simulink model "ramadan_2022"  (R2021a)
settings: Solver=ode15s  StartTime=0.0  StopTime=10  MaxStep=1e-2  MinStep=1e-20  RelTol=1e-3
StartFcn:
  | tic
StopFcn:
  | toc
  | 
  | 
  | %if GimbalLockFlag
  |  % fprintf(2, 'Almost reached Gimbal Lock of IMU. Simulation stopped.\n')
  | %end
  | 
  | %fprintf('Elapsed time: %4.2f sec (%4.2f%% realtime)\n', a, tout(end)/a*100)
values from neighbouring files (symbols this model uses):
  Balance = pMod(26:29)    [AssignSimulinkParams.m]    (also in assign_parameters.m = param(26:29))
  BalanceTrunkLat = pMod(22:25)    [AssignSimulinkParams.m]    (also in assign_parameters.m = param(22:25))
  BasisStim = pMod(1:11)    [AssignSimulinkParams.m]    (also in assign_parameters.m = param(1:11))
  CompliantLeg = pMod(12:14)    [AssignSimulinkParams.m]    (also in assign_parameters.m = param(12:14))
  CompliantLegLat = pMod(15)    [AssignSimulinkParams.m]    (also in assign_parameters.m = param(15))
  lp1 = 0.45    [nms3D_prep.m]
  lp2 = 0.55    [nms3D_prep.m]
  N = size(x,1)    [cmaes_hg.m]
  PreventKneeOverextension = pMod(16:21)    [AssignSimulinkParams.m]    (also in assign_parameters.m = param(16:21))
  propulsion = pMod(35)    [AssignSimulinkParams.m]    (also in assign_parameters.m = param(35))
  s = x(1:N-1,:).^2 + x(2:N,:).^2    [cmaes_hg.m]
  Target02 = pMod(30)    [AssignSimulinkParams.m]    (also in assign_parameters.m = param(30))
  Target13 = pMod(31:33)    [AssignSimulinkParams.m]    (also in assign_parameters.m = param(31:33))
  theta0 = pMod(34)    [AssignSimulinkParams.m]    (also in assign_parameters.m = param(34))
  WramameiSL_1000 = readmatrix('WSL_1000_Norm_Sigmoid_MSE_cont.csv')    [nms3D_prep.m]
  ZramameiSL_1000 = readmatrix('ZSL_1000_Norm_Sigmoid_MSE_cont.csv')    [nms3D_prep.m]
undefined symbols (not defined in the file or in its folder): ICs, mParams, X, Y, Z
libraries: nesl_utility x110, sm_lib x88, simulink x79, eeGeneralControl x28, robotmaniplib x10, dspinverses x10, robotcorelib x5, dspmathops x3, pid_lib x2, vrlib x1
(part 7 of 9)

== system ramadan_2022/Muscle Actuation Layer/Muscles Left/Muscle Torque Contributions1/Subsystem ==
  F VAS : Inport
  Moment Arm VAS : Inport  Port=2
  F SOL : Inport  Port=3
  Moment Arm SOL : Inport  Port=4
  Constant : Constant  Value=mParams.muscles.FmaxVec(7)
  Constant1 : Constant  Value=mParams.muscles.FmaxVec(10)
  Divide2 : Product  Inputs=*/
  Product{7..8,11..12} (4 alike) : Product
  Sum4 : Sum
  Sum6 : Sum
  "Leg Torque " : Outport
  wires:
  Sum4/1 -> Divide2/2
  Divide2/1 -> "Leg Torque "/1
  Moment Arm SOL/1 -> Product7/1, Product11/2
  Product11/1 -> Sum6/2
  Constant/1 -> Product8/2
  F VAS/1 -> Product12/1
  Moment Arm VAS/1 -> Product8/1, Product12/2
  Product7/1 -> Sum4/2
  F SOL/1 -> Product11/1
  Sum6/1 -> Divide2/1
  Product12/1 -> Sum6/1
  Constant1/1 -> Product7/2
  Product8/1 -> Sum4/1

== system ramadan_2022/Muscle Actuation Layer/Muscles Right/Muscle Dynamics (Vectorized)/BE force-length relation ==
  note: Buffer Elasticity BE
  lce [lopt] : Inport
  Constant1 : Constant  Value=1-mParams.muscles.w
  Math Function : Math  Operator=square  SignedPower=on  SaturateOnIntegerOverflow=on
  Sum4 : Sum  Inputs=|+-  InputSameDT=on  SaturateOnIntegerOverflow=on  OutDataTypeStr=Inherit: Same as first input
  buffer engaged? : simulink/Logic and Bit Operations/Compare To Zero  relop=<  OutDataTypeStr=boolean  ZeroCross=off
  force of buffer elasticity : Product  Inputs=**
  reference strain [lslack] : Constant  Value=mParams.muscles.w/2
  relative strain : Product  Inputs=*/
  fbe [Fmax] : Outport  VectorParamsAs1DForOutWhenUnconnected=off
  wires:
  force of buffer elasticity/1 -> fbe [Fmax]/1
  Math Function/1 -> force of buffer elasticity/2
  buffer engaged?/1 -> force of buffer elasticity/1
  Constant1/1 -> Sum4/2
  Sum4/1 -> relative strain/1, buffer engaged?/1
  reference strain [lslack]/1 -> relative strain/2
  relative strain/1 -> Math Function/1
  lce [lopt]/1 -> Sum4/1

== system ramadan_2022/Muscle Actuation Layer/Muscles Right/Muscle Dynamics (Vectorized)/CE force-length relation ==
  note: CE Force-Length Relationship
  lce [lopt] : Inport
  Abs : Abs  ZeroCross=off
  Constant1 : Constant
  Constant2 : Constant  Value=3
  Gain : Gain  Gain=log(mParams.muscles.c)
  Math Function : Math  SignedPower=on  SaturateOnIntegerOverflow=on
  Math Function1 : Math  Operator=pow  SignedPower=on  SaturateOnIntegerOverflow=on
  Sum4 : Sum  Inputs=|+-  InputSameDT=on  SaturateOnIntegerOverflow=on  OutDataTypeStr=Inherit: Same as first input
  normalized position : Product  Inputs=*/
  relative width : Constant  Value=mParams.muscles.w
  fce [Fmax] : Outport  VectorParamsAs1DForOutWhenUnconnected=off
  wires:
  Math Function/1 -> fce [Fmax]/1
  Gain/1 -> Math Function/1
  Math Function1/1 -> Gain/1
  Constant2/1 -> Math Function1/2
  normalized position/1 -> Math Function1/1
  Abs/1 -> normalized position/1
  Sum4/1 -> Abs/1
  Constant1/1 -> Sum4/2
  relative width/1 -> normalized position/2
  lce [lopt]/1 -> Sum4/1

== system ramadan_2022/Muscle Actuation Layer/Muscles Right/Muscle Dynamics (Vectorized)/CE inverse force-velocity relation ==
  note: CE Inverse Force-Velocity Relationship
  Fv[Fmax] : Inport
  1 : Product  Inputs=/*
  Constant{1,3..4,8} (4 alike) : Constant
  Constant2 : Constant  Value=mParams.muscles.N
  Curvature : Gain  Gain=mParams.muscles.K  SaturateOnIntegerOverflow=on  OutDataTypeStr=Inherit: Same as input  ParamDataTypeStr=Inherit: Same as input
  Curvature1 : Gain  Gain=7.56*mParams.muscles.K  SaturateOnIntegerOverflow=on  OutDataTypeStr=Inherit: Same as input  ParamDataTypeStr=Inherit: Same as input
  Logical Operator : Logic  Operator=NOT  AllPortsSameDT=off  OutDataTypeStr=boolean
  Logical Operator1 : Logic  Operator=NOT  AllPortsSameDT=off  OutDataTypeStr=boolean
  Slope : Gain  Gain=1e-2  SaturateOnIntegerOverflow=on  OutDataTypeStr=Inherit: Same as input  ParamDataTypeStr=Inherit: Same as input
  Sum1 : Sum  Inputs=|++  InputSameDT=on  SaturateOnIntegerOverflow=on  OutDataTypeStr=Inherit: Same as first input
  Sum2 : Sum  InputSameDT=on  SaturateOnIntegerOverflow=on  OutDataTypeStr=Inherit: Same as first input
  Sum3 : Sum  Inputs=++|  InputSameDT=on  SaturateOnIntegerOverflow=on  OutDataTypeStr=Inherit: Same as first input
  Sum4 : Sum  Inputs=|+-  InputSameDT=on  SaturateOnIntegerOverflow=on  OutDataTypeStr=Inherit: Same as first input
  Sum5 : Sum  Inputs=|-+  InputSameDT=on  SaturateOnIntegerOverflow=on  OutDataTypeStr=Inherit: Same as first input
  Sum6 : Sum  Inputs=-+|  InputSameDT=on  SaturateOnIntegerOverflow=on  OutDataTypeStr=Inherit: Same as first input
  Sum7 : Sum  Inputs=|++  InputSameDT=on  SaturateOnIntegerOverflow=on  OutDataTypeStr=Inherit: Same as first input
  Sum8 : Sum  Inputs=+-|  InputSameDT=on  SaturateOnIntegerOverflow=on  OutDataTypeStr=Inherit: Same as first input
  Sum9 : Sum  InputSameDT=on  SaturateOnIntegerOverflow=on  OutDataTypeStr=Inherit: Same as first input
  extension force within bound? : simulink/Logic and Bit Operations/Compare To Constant  relop=<=  const=mParams.muscles.N  OutDataTypeStr=boolean  ZeroCross=off
  force indicating contraction? : simulink/Logic and Bit Operations/Compare To Constant  relop=<=  const=1  OutDataTypeStr=boolean  ZeroCross=off
  v_concentric : Product  Inputs=*/
  v_concentric1 : Product  Inputs=**
  v_excentric <=N 1 : Product  Inputs=***
  v_excentric <N : Product  Inputs=*/
  v_excentric >N : Product  Inputs=**
  v[vmax] : Outport  VectorParamsAs1DForOutWhenUnconnected=off
  wires:
  Sum2/1 -> Sum9/2
  v_excentric <=N 1/1 -> Sum2/1
  Logical Operator1/1 -> v_excentric >N/1
  v_excentric >N/1 -> Sum2/2
  Logical Operator/1 -> v_excentric <=N 1/1
  Fv[Fmax]/1 -> extension force within bound?/1, force indicating contraction?/1, Curvature/1, Sum4/1, Sum6/2
  extension force within bound?/1 -> Logical Operator1/1, v_excentric <=N 1/3
  force indicating contraction?/1 -> Logical Operator/1, v_concentric1/2
  Sum1/1 -> v_excentric >N/2
  v_concentric1/1 -> Sum9/1
  v_excentric <N/1 -> v_excentric <=N 1/2
  Constant3/1 -> Sum5/1
  Sum5/1 -> 1/1
  Constant2/1 -> Sum5/2, Sum6/1
  Sum6/1 -> Slope/1, 1/2
  Constant8/1 -> Sum1/2
  Slope/1 -> Sum1/1
  Sum9/1 -> v[vmax]/1
  v_concentric/1 -> v_concentric1/1
  Sum7/1 -> v_excentric <N/1
  Sum8/1 -> v_excentric <N/2
  Curvature1/1 -> Sum8/2
  Constant4/1 -> Sum8/1, Sum7/2
  1/1 -> Curvature1/1, Sum7/1
  Sum3/1 -> v_concentric/2
  Sum4/1 -> v_concentric/1
  Constant1/1 -> Sum3/1, Sum4/2
  Curvature/1 -> Sum3/2

== system ramadan_2022/Muscle Actuation Layer/Muscles Right/Muscle Dynamics (Vectorized)/PE force-length relation ==
  note: Parallel Elasticity PE
  lce [lopt] : Inport
  Constant3 : Constant
  Math Function2 : Math  Operator=square  SignedPower=on  SaturateOnIntegerOverflow=on
  Sum1 : Sum  Inputs=|+-  InputSameDT=on  SaturateOnIntegerOverflow=on  OutDataTypeStr=Inherit: Same as first input
  force of buffer elasticity : Product  Inputs=**
  parallel elasticity engaged? : simulink/Logic and Bit Operations/Compare To Zero  relop=>  OutDataTypeStr=boolean  ZeroCross=off
  reference strain [lopt] : Constant  Value=mParams.muscles.w
  relative strain : Product  Inputs=*/
  fpe [Fmax] : Outport  VectorParamsAs1DForOutWhenUnconnected=off
  wires:
  parallel elasticity engaged?/1 -> force of buffer elasticity/1
  force of buffer elasticity/1 -> fpe [Fmax]/1
  Math Function2/1 -> force of buffer elasticity/2
  relative strain/1 -> Math Function2/1
  reference strain [lopt]/1 -> relative strain/2
  Sum1/1 -> relative strain/1, parallel elasticity engaged?/1
  Constant3/1 -> Sum1/2
  lce [lopt]/1 -> Sum1/1

== system ramadan_2022/Muscle Actuation Layer/Muscles Right/Muscle Dynamics (Vectorized)/SE force-length relation ==
  note: SE Force-Length Relationship
  lse [lslack] : Inport
  Constant1 : Constant
  Math Function : Math  Operator=square  SignedPower=on  SaturateOnIntegerOverflow=on
  Sum4 : Sum  Inputs=|+-  InputSameDT=on  SaturateOnIntegerOverflow=on  OutDataTypeStr=Inherit: Same as first input
  force above slack length : Product  Inputs=**
  greater than slack length? : simulink/Logic and Bit Operations/Compare To Zero  relop=>  OutDataTypeStr=boolean  ZeroCross=off
  reference strain [lslack] : Constant  Value=mParams.muscles.eref
  relative strain : Product  Inputs=*/
  fse [Fmax] : Outport  VectorParamsAs1DForOutWhenUnconnected=off
  wires:
  force above slack length/1 -> fse [Fmax]/1
  greater than slack length?/1 -> force above slack length/1
  Constant1/1 -> Sum4/2
  Sum4/1 -> relative strain/1, greater than slack length?/1
  relative strain/1 -> Math Function/1
  lse [lslack]/1 -> Sum4/1
  Math Function/1 -> force above slack length/2
  reference strain [lslack]/1 -> relative strain/2

== system ramadan_2022/Muscle Actuation Layer/Muscles Right/Muscle Torque Contributions/Subsystem ==
  F VAS : Inport
  Moment Arm VAS : Inport  Port=2
  F SOL : Inport  Port=3
  Moment Arm SOL : Inport  Port=4
  Constant : Constant  Value=mParams.muscles.FmaxVec(7)
  Constant1 : Constant  Value=mParams.muscles.FmaxVec(10)
  Divide2 : Product  Inputs=*/
  Product{7..8,11..12} (4 alike) : Product
  Sum4 : Sum
  Sum6 : Sum
  "Leg Torque " : Outport
  wires:
  Sum4/1 -> Divide2/2
  Divide2/1 -> "Leg Torque "/1
  Moment Arm SOL/1 -> Product7/1, Product11/2
  Product11/1 -> Sum6/2
  Constant/1 -> Product8/2
  F VAS/1 -> Product12/1
  Moment Arm VAS/1 -> Product8/1, Product12/2
  Product7/1 -> Sum4/2
  F SOL/1 -> Product11/1
  Sum6/1 -> Divide2/1
  Product12/1 -> Sum6/1
  Constant1/1 -> Product7/2
  Product8/1 -> Sum4/1

== system ramadan_2022/Supraspinal Level/Subsystem/Compute positives forces that generate desired torque profiles/Left ==
  Desired Torques : Inport
  Angles : Inport  Port=2
  Constant : Constant  Value=WramameiSL_1000  VectorParams1D=off  SampleTime=-1
  Constant1 : Constant  Value=|
      | [1.666708374023437500e+01
      | -3.333266830444335938e+01]
  Constant2 : Constant  Value=ZramameiSL_1000
  Denorm : Gain  Gain=[2000, 1500, 3000, 1200, 6000, 350, 1500, 4000, 800]
  Matrix Concatenate : Concatenate  Mode=Multidimensional array
  Matrix Concatenate4 : Concatenate  Mode=Multidimensional array  ConcatenateDimension=2
  Matrix Multiply2 : Product  Multiplication=Matrix(*)
  Matrix Multiply3 : Product  Multiplication=Matrix(*)
  Matrix Multiply8 : Product  Multiplication=Matrix(*)
  Multiply : Gain  Gain=1/960
  Multiply2 : Gain  Gain=1/3.0543
  Saturation : Saturate  UpperLimit=inf  LowerLimit=0  ZeroCross=off
  Saturation2 : Saturate  UpperLimit=inf  LowerLimit=0  ZeroCross=off
  Selector : Selector  InputPortWidth=4  IndexOptions=Index vector (dialog)  Indices=[1 3 4]  OutputSizes=1
  Selector1 : Selector  InputPortWidth=4  IndexOptions=Index vector (dialog)  Indices=[3 4]  OutputSizes=1
  Selector8 : Selector  InputPortWidth=4  IndexOptions=Index vector (dialog)  Indices=2  OutputSizes=1
  Transpose3 : Math  Operator=transpose  SaturateOnIntegerOverflow=on
  Transpose9 : Math  Operator=transpose  SaturateOnIntegerOverflow=on
  sigmoid : Subsystem
  Forces : Outport
  wires:
  Desired Torques/1 -> Selector/1, Selector8/1
  Selector1/1 -> Multiply2/1
  Matrix Multiply2/1 -> Saturation/1
  Selector/1 -> Multiply/1
  Constant/1 -> Matrix Multiply3/2
  Constant2/1 -> Matrix Multiply2/2
  Angles/1 -> Selector1/1
  Matrix Multiply8/1 -> Saturation2/1
  Constant1/1 -> Transpose9/1
  Selector8/1 -> Matrix Multiply8/1
  Transpose9/1 -> Matrix Multiply8/2
  Saturation/1 -> Denorm/1
  Matrix Concatenate4/1 -> Forces/1
  Saturation2/1 -> Matrix Concatenate4/1
  Transpose3/1 -> Matrix Multiply3/1
  Matrix Concatenate/1 -> Transpose3/1  "tr"
  Denorm/1 -> Matrix Concatenate4/2
  Multiply/1 -> Matrix Concatenate/1
  Multiply2/1 -> Matrix Concatenate/2
  sigmoid/1(Out1) -> Matrix Multiply2/1
  Matrix Multiply3/1 -> sigmoid/1(In1)

== system ramadan_2022/Supraspinal Level/Subsystem/Compute positives forces that generate desired torque profiles/Right ==
  Desired Torques : Inport
  Angles : Inport  Port=2
  Constant : Constant  Value=WramameiSL_1000  VectorParams1D=off  SampleTime=-1
  Constant1 : Constant  Value=|
      | [1.666708374023437500e+01
      | -3.333266830444335938e+01]
  Constant2 : Constant  Value=ZramameiSL_1000
  Denorm : Gain  Gain=[2000, 1500, 3000, 1200, 6000, 350, 1500, 4000, 800]
  Matrix Concatenate : Concatenate  Mode=Multidimensional array
  Matrix Concatenate4 : Concatenate  Mode=Multidimensional array  ConcatenateDimension=2
  Matrix Multiply2 : Product  Multiplication=Matrix(*)
  Matrix Multiply3 : Product  Multiplication=Matrix(*)
  Matrix Multiply8 : Product  Multiplication=Matrix(*)
  Multiply : Gain  Gain=1/960
  Multiply2 : Gain  Gain=1/3.0543
  Saturation : Saturate  UpperLimit=inf  LowerLimit=0  ZeroCross=off
  Saturation2 : Saturate  UpperLimit=inf  LowerLimit=0  ZeroCross=off
  Selector : Selector  InputPortWidth=4  IndexOptions=Index vector (dialog)  Indices=[1 3 4]  OutputSizes=1
  Selector1 : Selector  InputPortWidth=4  IndexOptions=Index vector (dialog)  Indices=[3 4]  OutputSizes=1
  Selector8 : Selector  InputPortWidth=4  IndexOptions=Index vector (dialog)  Indices=2  OutputSizes=1
  Transpose3 : Math  Operator=transpose  SaturateOnIntegerOverflow=on
  Transpose9 : Math  Operator=transpose  SaturateOnIntegerOverflow=on
  sigmoid : Subsystem
  Forces : Outport
  wires:
  Desired Torques/1 -> Selector/1, Selector8/1
  Selector1/1 -> Multiply2/1
  Matrix Multiply2/1 -> Saturation/1
  Selector/1 -> Multiply/1
  Constant/1 -> Matrix Multiply3/2
  Constant2/1 -> Matrix Multiply2/2
  Angles/1 -> Selector1/1
  Matrix Multiply8/1 -> Saturation2/1
  Constant1/1 -> Transpose9/1
  Selector8/1 -> Matrix Multiply8/1
  Transpose9/1 -> Matrix Multiply8/2
  Saturation/1 -> Denorm/1
  Matrix Concatenate4/1 -> Forces/1
  Saturation2/1 -> Matrix Concatenate4/1
  Transpose3/1 -> Matrix Multiply3/1
  Matrix Concatenate/1 -> Transpose3/1  "tr"
  Denorm/1 -> Matrix Concatenate4/2
  Multiply/1 -> Matrix Concatenate/1
  Multiply2/1 -> Matrix Concatenate/2
  sigmoid/1(Out1) -> Matrix Multiply2/1
  Matrix Multiply3/1 -> sigmoid/1(In1)

== system ramadan_2022/Supraspinal Level/Subsystem/Stance Leg2/Balance Control Equation [Ankle Strategy] ==
  Desired Acceleration (CoM) : Outport
  wires:
  [propulsion] -> Desired Acceleration (CoM)/1

== system ramadan_2022/Supraspinal Level/Subsystem/Stance Leg2/PD-Controller For Saggital Trunk Balance ==
  Gain : Gain  Gain=-1
  Gain1 : Gain  Gain=-1
  Low-Pass Filter (Discrete or Continuous) : eeGeneralControl/Low-Pass Filter (Discrete or Continuous)  K=1  T=0.01  B=inf  A=-inf  init_option=Inherited from block input  x0=0  Ts=0
  Minus : Sum  Inputs=+-
  PID Controller : pid_lib/PID Controller  Controller=PD  Form=Parallel  TimeDomain=Continuous-time  UseExternalTs=off  SampleTime=-1  IntegratorMethod=Forward Euler  FilterMethod=Forward Euler  ControllerParametersSource=internal  P=30  I=0  D=80  UseFilter=on  N=100  TunerSelectOption=Transfer Function Based (PID Tuner App)  ZeroCross=off  InitialConditionSource=internal  InitialConditionForIntegrator=0  InitialConditionForFilter=0  DifferentiatorICPrevScaledInput=0  ExternalReset=none  TrackingMode=off  Kt=1  LimitOutput=off  SatLimitsSource=internal  UpperSaturationLimit=inf  LowerSaturationLimit=-inf  LinearizeAsGain=on  AntiWindupMode=none  Kb=1  POutMin=[]  POutMax=[]  IOutMin=[]  IOutMax=[]  DOutMin=[]  DOutMax=[]  NOutMin=[]  NOutMax=[]  SumOutMin=[]  SumOutMax=[]  SaturationOutMin=[]  SaturationOutMax=[]  PParamMin=[]  PParamMax=[]  IParamMin=[]  IParamMax=[]  DParamMin=[]  DParamMax=[]  NParamMin=[]  NParamMax=[]  KbParamMin=[]  KbParamMax=[]  KtParamMin=[]  KtParamMax=[]  KbOutMin=[]  KbOutMax=[]  KtOutMin=[]  KtOutMax=[]  IntegratorOutMin=[]  IntegratorOutMax=[]  FilterOutMin=[]  FilterOutMax=[]  SumI1OutMin=[]  SumI1OutMax=[]  SumI2OutMin=[]  SumI2OutMax=[]  SumI3OutMin=[]  SumI3OutMax=[]  SumI4OutMin=[]  SumI4OutMax=[]  SumDOutMin=[]  SumDOutMax=[]  DifferentiatorOutMin=[]  DifferentiatorOutMax=[]  FilterDiffOutCoefMin=[]  FilterDiffOutCoefMax=[]  ReciprocalOutMin=[]  ReciprocalOutMax=[]  SumDenOutMin=[]  SumDenOutMax=[]  SumNumOutMin=[]  SumNumOutMax=[]  DivideOutMin=[]  DivideOutMax=[]  UdiffTsProdOutMin=[]  UdiffTsProdOutMax=[]  NTsProdOutMin=[]  NTsProdOutMax=[]  UintegralTsProdOutMin=[]  UintegralTsProdOutMax=[]  UngainTsProdOutMin=[]  UngainTsProdOutMax=[]  IntegratorContinuousStateAttributes=''  IntegratorStateMustResolveToSignalObject=off  IntegratorRTWStateStorageClass=Auto  FilterContinuousStateAttributes=''  FilterStateMustResolveToSignalObject=off  FilterRTWStateStorageClass=Auto  ParallelPVariant=InternalParameters  IdealPVariant=Disabled  IVariant=Disabled  DVariant=InternalParameters  IntegratorVariant=Disabled  SatVariant=Disabled  AWVariant=Disabled  PCopyVariant=Disabled  TRVariant=Disabled  FdbkBlocksVariant=Forward  IdealPFdbkVariant=Disabled  SatFdbkVariant=Disabled  DerivativeFilterVariant=ContFilter  NVariant=InternalParameters  NCopyVariant=Disabled  FilterICVariant=InternalICsFilter  IntegratorICVariant=Disabled  ExternalResetVariant=Disabled  TRSumVariant=Passthrough  SumFdbkVariant=Disabled  SumVariant=Sum_PD  TsampFilterVariant=InternalTs  TsampNgainVariant=Passthrough  TsampIntegralVariant=Disabled_SignalSpec  ExternalSaturationOutDataTypeStr=Inherit: Same as second input
  To Workspace6 : ToWorkspace  VariableName=RotSag  SampleTime=-1
      settings: Save2DSignal=2-D array (concatenate along first dimension)
  PD Input : Outport
  wires:
  Gain/1 -> Low-Pass Filter (Discrete or Continuous)/1
  Minus/1 -> PID Controller/1
  [TrunkRot_sag] -> To Workspace6/1, Minus/1
  PID Controller/1 -> Gain/1
  [theta0] -> Gain1/1
  Gain1/1 -> Minus/2
  Low-Pass Filter (Discrete or Continuous)/1 -> PD Input/1

== system ramadan_2022/Supraspinal Level/Subsystem/Stance Leg2/Stance Leg ==
  left/right : Inport
  Balance Control [Ankle Strategy] : Inport  Port=2
  PD Input : Inport  Port=3
  Foot Orientation Left : Subsystem
  Foot Orientation Right : Subsystem
  Inverse Dynamics Left Leg : Subsystem
  Mux : Mux  Inputs=2
  Mux1 : Mux  Inputs=2
  NOT2 : Logic  Operator=NOT  AllPortsSameDT=off  OutDataTypeStr=boolean
  Selector : Selector  InputPortWidth=4  IndexOptions=Index vector (dialog)  Indices=[ 4 3 2 1]  OutputSizes=1
  Selector1 : Selector  InputPortWidth=4  IndexOptions=Index vector (dialog)  Indices=[ 4 3 2 1]  OutputSizes=1
  Subsystem : Subsystem
  Transpose : Math  Operator=transpose  SaturateOnIntegerOverflow=on
  long delay 1 : eeGeneralControl/Low-Pass Filter (Discrete or Continuous)  K=1  T=mParams.control.delays.long  B=inf  A=-inf  init_option=Inherited from block input  x0=0  Ts=-1
  long delay 2 : eeGeneralControl/Low-Pass Filter (Discrete or Continuous)  K=1  T=mParams.control.delays.long  B=inf  A=-inf  init_option=Inherited from block input  x0=0  Ts=-1
  long delay 4 : eeGeneralControl/Low-Pass Filter (Discrete or Continuous)  K=1  T=mParams.control.delays.long  B=inf  A=-inf  init_option=Inherited from block input  x0=0  Ts=-1
  Push Off Left : Outport
  Push-Off Right : Outport  Port=2
  wires:
  [Rlegq] -> long delay 2/1
  Selector/1 -> Mux/2
  Selector1/1 -> Mux1/2
  [R_body] -> long delay 4/1
  left/right/1 -> NOT2/1, Inverse Dynamics Left Leg/2(left/right)
  Transpose/1 -> Foot Orientation Right/1(R Pelvis), Foot Orientation Left/1(R Pelvis)
  Foot Orientation Left/1(Orientation Foot (Z)) -> Mux1/1
  Foot Orientation Right/1(Foot Orientation (Z)) -> Mux/1
  Balance Control [Ankle Strategy]/1 -> Inverse Dynamics Left Leg/3(Task), Subsystem/3(Task)
  Inverse Dynamics Left Leg/1(Push-Off (Left)) -> Push Off Left/1
  Mux/1 -> Subsystem/1(Config [5])
  NOT2/1 -> Subsystem/2(left/right)
  Subsystem/1(Push-Off (Right)) -> Push-Off Right/1
  Mux1/1 -> Inverse Dynamics Left Leg/1(Config [5])
  long delay 1/1 -> Selector1/1
  long delay 2/1 -> Selector/1
  long delay 4/1 -> Transpose/1
  [Llegq] -> long delay 1/1
  PD Input/1 -> Subsystem/4(PD Input), Inverse Dynamics Left Leg/4(PD Input)

== system ramadan_2022/Supraspinal Level/Subsystem/Swing Leg/Check Quality Minimal Jerk ==
  In1 : Inport
  In2 : Inport  Port=2
  In3 : Inport  Port=3
  In4 : Inport  Port=4
  Mux1 : Mux
  Mux2 : Mux
  Scope : Scope  NumInputPorts=2
  Scope1 : Scope  NumInputPorts=2
  Selector{1..4} (4 alike) : Selector  InputPortWidth=3  IndexOptions=Index vector (dialog)  Indices=[ 3]  OutputSizes=1
  Selector{5..8} (4 alike) : Selector  InputPortWidth=3  IndexOptions=Index vector (dialog)  Indices=[ 1]  OutputSizes=1
  wires:
  Selector5/1 -> Mux2/1
  Selector1/1 -> Mux1/1
  Mux2/1 -> Scope1/2
  Mux1/1 -> Scope/2
  In1/1 -> Selector5/1, Selector1/1
  Selector8/1 -> Mux2/4
  [Rlegddq] -> Scope/1
  Selector3/1 -> Mux1/3
  Selector2/1 -> Mux1/2
  Selector6/1 -> Mux2/2
  In4/1 -> Selector6/1, Selector2/1
  In3/1 -> Selector4/1, Selector8/1
  In2/1 -> Selector3/1, Selector7/1
  [Rlegq] -> Scope1/1
  Selector7/1 -> Mux2/3
  Selector4/1 -> Mux1/4

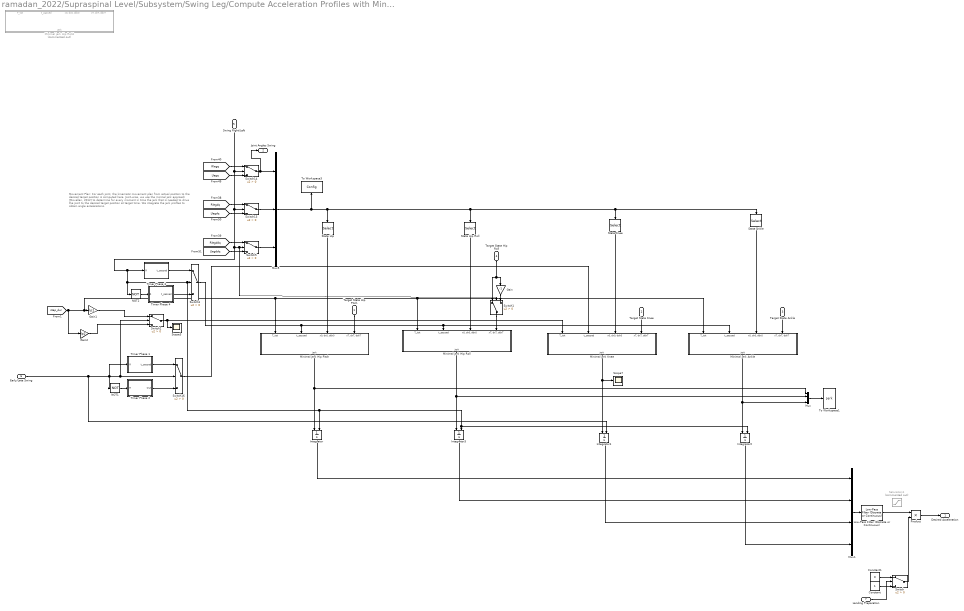
== system ramadan_2022/Supraspinal Level/Subsystem/Swing Leg/Compute Acceleration Profiles with Minimal Jerk Approach ==
  note: Movement Plan: For each joint, the kinematic movement plan from actual position to the desired target position is computed here. Joint-wise, we use the mininal jerk approach [Movellan, 2012] to determine for every moment in time the jerk that is needed to drive the joint to the desired target position at target time. We integrate the jerk profiles to obtain angle accelerations.
  Target State Hip Pitch : Inport
  Target State Knee : Inport  Port=2
  Target State Ankle : Inport  Port=3
  Target State Hip Roll : Inport  Port=4
  Swing Right/Left : Inport  Port=5
  Early/Late Swing : Inport  Port=6
  Landing Preparation : Inport  Port=7
  " Timer Phase 1" : Subsystem
  " Timer Phase 2" : Subsystem
  " Timer Phase 3" : Subsystem
  " Timer Phase 4" : Subsystem
  Constant : Constant
  Constant1 : Constant  Value=0
  Gain : Gain  Gain=-1
  Gain1 : Gain  Gain=lp1
  Gain2 : Gain  Gain=lp2
  Integrator{,1..3} (4 alike) : Integrator  ExternalReset=either  ZeroCross=off
  Low-Pass Filter (Discrete or Continuous) : eeGeneralControl/Low-Pass Filter (Discrete or Continuous)  K=1  T=0.001  B=2000  A=-2000  init_option=Inherited from block input  x0=0  Ts=0
  Minimal jerk Ankle : Subsystem
  Minimal jerk Hip Pitch : Subsystem
  Minimal jerk Hip Roll : Subsystem
  Minimal jerk Hip Roll4 : Subsystem  Commented=on
  Minimal jerk Knee : Subsystem
  Mux : Mux
  Mux1 : Mux
  Mux5 : Mux  Inputs=3
  NOT1 : Logic  Operator=NOT  AllPortsSameDT=off  OutDataTypeStr=boolean
  NOT2 : Logic  Operator=NOT  AllPortsSameDT=off  OutDataTypeStr=boolean
  Product : Product
  Saturation1 : Saturate  Commented=on  UpperLimit=2000  LowerLimit=-2000  ZeroCross=off
  Scope3 : Scope
  Scope7 : Scope
  State Ankle : Selector  InputPortWidth=12  IndexOptions=Index vector (dialog)  Indices=[4 8 12]  OutputSizes=1
  State Hip : Selector  InputPortWidth=12  IndexOptions=Index vector (dialog)  Indices=[1 5 9]  OutputSizes=1
  State Hip Roll : Selector  InputPortWidth=12  IndexOptions=Index vector (dialog)  Indices=[2 6 10 ]  OutputSizes=1
  State Knee : Selector  InputPortWidth=12  IndexOptions=Index vector (dialog)  Indices=[3 7 11 ]  OutputSizes=1
  Switch : Switch  Criteria=u2 > Threshold  ZeroCross=off
  Switch{1..3,5,13..14,16} (7 alike) : Switch  Criteria=u2 > Threshold
  To Workspace1 : ToWorkspace  VariableName=Jerk  SampleTime=-1
      settings: Save2DSignal=2-D array (concatenate along first dimension)
  To Workspace3 : ToWorkspace  VariableName=Config  SampleTime=-1
      settings: Save2DSignal=2-D array (concatenate along first dimension)
  "Desired Acceleration " : Outport
  Joint Angles Swing : Outport  Port=2
  wires:
  State Hip/1 -> Minimal jerk Hip Pitch/3("x0, dx0, ddx0")
  NOT1/1 -> " Timer Phase 2"/1(R)
  Mux1/1 -> Low-Pass Filter (Discrete or Continuous)/1
  Switch2/1 -> Scope3/1, Minimal jerk Knee/1(T_tot)
  [Llegddq] -> Switch5/3
  [Rlegq] -> Switch14/1
  [Llegdq] -> Switch13/3
  Target State Hip Pitch/1 -> Minimal jerk Hip Pitch/4("xT, dxT, ddxT")
  Target State Knee/1 -> Minimal jerk Knee/4("xT, dxT, ddxT")
  [Rlegddq] -> Switch5/1
  Integrator1/1 -> Mux1/3
  Switch5/1 -> Mux5/3
  [Llegq] -> Switch14/3
  State Knee/1 -> Minimal jerk Knee/3("x0, dx0, ddx0")
  Target State Ankle/1 -> Minimal jerk Ankle/4("xT, dxT, ddxT")
  Integrator/1 -> Mux1/1
  Switch14/1 -> Joint Angles Swing/1, Mux5/1
  Integrator2/1 -> Mux1/4
  State Ankle/1 -> Minimal jerk Ankle/3("x0, dx0, ddx0")
  Switch13/1 -> Mux5/2
  [Rlegdq] -> Switch13/1
  Early/Late Swing/1 -> Switch2/2, Switch16/2, NOT1/1, " Timer Phase 1"/1(R), Integrator1/2
  Swing Right/Left/1 -> Switch14/2, Switch13/2, NOT2/1, Integrator2/2, Integrator3/2, Integrator/2, Switch3/2, " Timer Phase 3"/1(R), Switch1/2, Switch5/2
  Switch16/1 -> Minimal jerk Knee/2(t_passed)
  State Hip Roll/1 -> Minimal jerk Hip Roll/3("x0, dx0, ddx0")
  Integrator3/1 -> Mux1/2
  Switch1/1 -> Minimal jerk Hip Roll/4("xT, dxT, ddxT")
  Target State Hip Roll/1 -> Gain/1, Switch1/1
  Gain/1 -> Switch1/3
  [step_dur] -> Gain2/1, Minimal jerk Hip Pitch/1(T_tot), Minimal jerk Hip Roll/1(T_tot), Minimal jerk Ankle/1(T_tot), Gain1/1
  " Timer Phase 1"/1(t_passed) -> Switch16/1
  " Timer Phase 2"/1(Out) -> Switch16/3
  Mux5/1 -> State Hip Roll/1, State Ankle/1, State Knee/1, State Hip/1, To Workspace3/1
  Mux/1 -> To Workspace1/1
  Minimal jerk Hip Pitch/1(jerk) -> Mux/1, Integrator/1
  Minimal jerk Hip Roll/1(jerk) -> Mux/2, Integrator3/1
  Minimal jerk Knee/1(jerk) -> Scope7/1, Integrator1/1
  Minimal jerk Ankle/1(jerk) -> Mux/4, Integrator2/1
  Low-Pass Filter (Discrete or Continuous)/1 -> Product/1
  Constant/1 -> Switch/3
  Constant1/1 -> Switch/1
  Switch/1 -> Product/2
  Product/1 -> "Desired Acceleration "/1
  Gain1/1 -> Switch2/1
  Gain2/1 -> Switch2/3
  NOT2/1 -> " Timer Phase 4"/1(R)
  " Timer Phase 3"/1(t_passed) -> Switch3/1
  " Timer Phase 4"/1(t_passed) -> Switch3/3
  Switch3/1 -> Minimal jerk Hip Pitch/2(t_passed), Minimal jerk Ankle/2(t_passed), Minimal jerk Hip Roll/2(t_passed)
  Landing Preparation/1 -> Switch/2

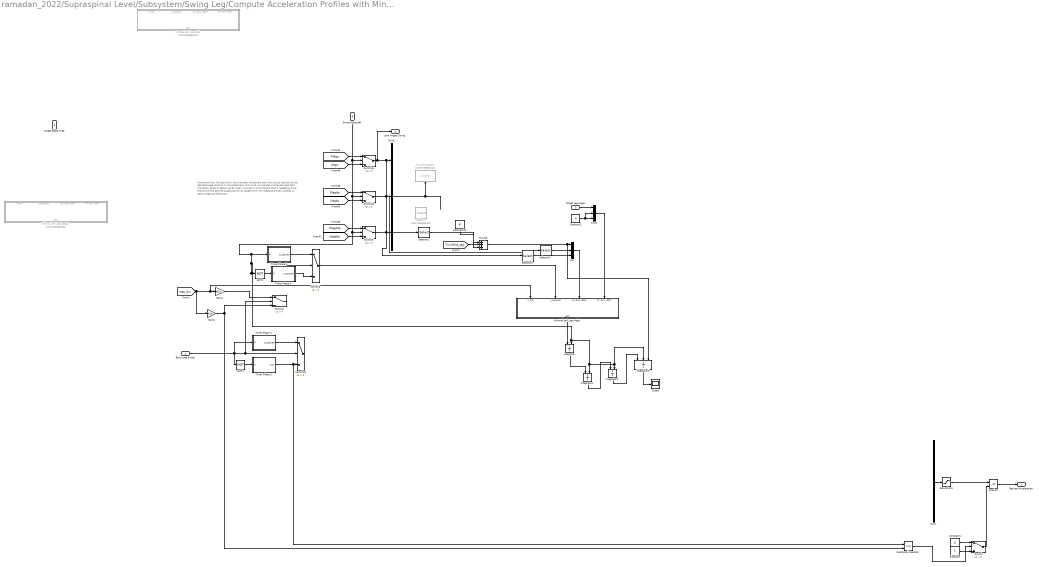
== system ramadan_2022/Supraspinal Level/Subsystem/Swing Leg/Compute Acceleration Profiles with Minimal Jerk Approach1 ==
  note: Movement Plan: For each joint, the kinematic movement plan from actual position to the desired target position is computed here. Joint-wise, we use the mininal jerk approach [Movellan, 2012] to determine for every moment in time the jerk that is needed to drive the joint to the desired target position at target time. We integrate the jerk profiles to obtain angle accelerations.
  Target Leg Angle : Inport
  Target State Knee : Inport  Port=2
  Swing Right/Left : Inport  Port=3
  Early/Late Swing : Inport  Port=4
  " Timer Phase 1" : Subsystem
  " Timer Phase 2" : Subsystem
  " Timer Phase 3" : Subsystem
  " Timer Phase 4" : Subsystem
  Constant : Constant
  Constant1 : Constant  Value=0
  Constant13 : Constant  Value=pi
  Constant2 : Constant  Value=0
  Gain1 : Gain  Gain=6/10
  Gain2 : Gain  Gain=4/10
  Integrator : Integrator  ExternalReset=either  ZeroCross=off
  Integrator1 : Integrator  ExternalReset=either  ZeroCross=off
  Integrator2 : Integrator  ExternalReset=either  ZeroCross=off
  Integrator3 : Integrator  ExternalReset=either  InitialConditionSource=external  ZeroCross=off
  Minimal jerk Hip Roll4 : Subsystem  Commented=on
  Minimal jerk Leg Angle : Subsystem
  Minimal jerk Leg Length : Subsystem  Commented=on
  Minus8 : Sum  Inputs=+++
  Mux : Mux  Inputs=3
  Mux1 : Mux
  Mux2 : Mux  Inputs=3
  Mux5 : Mux  Inputs=3
  NOT1 : Logic  Operator=NOT  AllPortsSameDT=off  OutDataTypeStr=boolean
  NOT2 : Logic  Operator=NOT  AllPortsSameDT=off  OutDataTypeStr=boolean
  Product : Product
  Relational Operator : RelationalOperator  OutDataTypeStr=boolean  ZeroCross=off  RndMeth=Simplest
  Saturation1 : Saturate  UpperLimit=2000  LowerLimit=-2000  ZeroCross=off
  Scope : Scope
  Selector : Selector  Commented=on  InputPortWidth=4  IndexOptions=Index vector (dialog)  Indices=[1]  OutputSizes=1
  Selector1 : Selector  InputPortWidth=4  IndexOptions=Index vector (dialog)  Indices=[1]  OutputSizes=1
  Selector2 : Selector  InputPortWidth=4  IndexOptions=Index vector (dialog)  Indices=[1]  OutputSizes=1
  Selector3 : Selector  InputPortWidth=4  IndexOptions=Index vector (dialog)  Indices=[1]  OutputSizes=1
  Switch{,2..3,5,13..14,16} (7 alike) : Switch  Criteria=u2 > Threshold
  To Workspace3 : ToWorkspace  Commented=on  VariableName=Config  SampleTime=-1
      settings: Save2DSignal=2-D array (concatenate along first dimension)
  "Desired Acceleration " : Outport
  Joint Angles Swing : Outport  Port=2
  wires:
  NOT1/1 -> " Timer Phase 2"/1(R)
  Mux1/1 -> Saturation1/1
  [Llegddq] -> Switch5/3
  [Rlegq] -> Switch14/1
  [Llegdq] -> Switch13/3
  [Rlegddq] -> Switch5/1
  Switch5/1 -> Selector3/1, Mux5/3
  [Llegq] -> Switch14/3
  Switch14/1 -> Joint Angles Swing/1, Selector1/1, Mux5/1
  Switch13/1 -> Selector2/1, Mux5/2
  [Rlegdq] -> Switch13/1
  Early/Late Swing/1 -> Switch2/2, Switch16/2, NOT1/1, " Timer Phase 1"/1(R)
  Swing Right/Left/1 -> Switch14/2, Switch13/2, Integrator3/2, Integrator2/2, Integrator1/2, Integrator/2, Switch3/2, NOT2/1, " Timer Phase 3"/1(R), Switch5/2
  [step_dur] -> Gain2/1, Minimal jerk Leg Angle/1(T_tot), Gain1/1
  " Timer Phase 1"/1(t_passed) -> Switch16/1
  " Timer Phase 2"/1(Out) -> Relational Operator/1, Switch16/3
  Mux5/1 -> To Workspace3/1
  Saturation1/1 -> Product/1
  Relational Operator/1 -> Switch/2
  Constant/1 -> Switch/3
  Constant1/1 -> Switch/1
  Switch/1 -> Product/2
  Product/1 -> "Desired Acceleration "/1
  Gain1/1 -> Switch2/1
  Gain2/1 -> Switch2/3, Relational Operator/2
  NOT2/1 -> " Timer Phase 4"/1(R)
  " Timer Phase 3"/1(t_passed) -> Switch3/1
  " Timer Phase 4"/1(t_passed) -> Switch3/3
  Switch3/1 -> Minimal jerk Leg Angle/2(t_passed)
  Mux/1 -> Minimal jerk Leg Angle/3("x0, dx0, ddx0")
  Mux2/1 -> Minimal jerk Leg Angle/4("xT, dxT, ddxT")
  Target Leg Angle/1 -> Mux2/1
  Constant2/1 -> Mux2/2, Mux2/3
  [TrunkRot_sag] -> Minus8/2
  Constant13/1 -> Minus8/1
  Minus8/1 -> Integrator3/3, Mux/1
  Minimal jerk Leg Angle/1(jerk) -> Integrator/1
  Integrator/1 -> Integrator1/1
  Selector1/1 -> Minus8/3
  Selector2/1 -> Mux/2
  Selector3/1 -> Mux/3
  Integrator1/1 -> Integrator2/1
  Integrator2/1 -> Integrator3/1
  Integrator3/1 -> Scope/1

== system ramadan_2022/Supraspinal Level/Subsystem/Swing Leg/Compute Target States ==
  note: Target Joint States: Target joint angles, angle velocities and angle acceleration are defined here. For knee and ankle, values are constant. For hip pitch and hip roll, values are computed using the Balance Control mechanism from [Yin et. al. 2007].
      | Low pass filters are added here to compensate for abrupt changes in target angles at transitions between early and late swing.
  Left/Right : Inport
  early/late : Inport  Port=2
  Balance Control lateral : Subsystem
  Balance Control saggital : Subsystem
  Constant : Constant  Value=0
  Constant1 : Constant  Value=50
  Constant13 : Constant  Value=pi
  Constant2 : Constant  Value=-150
  Constant3 : Constant  Value=-20
  Gain3 : Gain  Gain=-1
  Low-Pass Filter (Discrete or Continuous)1 : eeGeneralControl/Low-Pass Filter (Discrete or Continuous)  K=1  T=0.1  B=inf  A=-inf  init_option=Inherited from block input  x0=-13  Ts=-1
  Low-Pass Filter (Discrete or Continuous)2 : eeGeneralControl/Low-Pass Filter (Discrete or Continuous)  K=1  T=0.1  B=inf  A=-inf  init_option=Inherited from block input  x0=-13  Ts=-1
  Minus1 : Sum
  Minus8 : Sum  Inputs=+++
  Mux{2..3,5..6} (4 alike) : Mux  Inputs=3
  Product : Product
  Scope : Scope
  Sign : Signum  ZeroCross=off
  Switch : Switch  Criteria=u2 > Threshold
  Hip Pitch Target : Outport
  Knee Target : Outport  Port=2
  Ankle Target : Outport  Port=3
  Hip Roll Target : Outport  Port=4
  wires:
  [TrunkRot_sag] -> Scope/1, Minus8/3
  Left/Right/1 -> Balance Control lateral/1(Left/Right), Balance Control saggital/1(Left/Right)
  Gain3/1 -> Minus8/1
  [swk] -> Mux5/1
  Balance Control lateral/1(theta_Hip_swing_target) -> Sign/1, Minus1/1
  Balance Control saggital/1(theta_Hip_swing_target) -> Gain3/1
  Mux5/1 -> Knee Target/1
  Constant13/1 -> Minus8/2
  [TrunkRot_lat] -> Minus1/2
  Mux2/1 -> Low-Pass Filter (Discrete or Continuous)2/1
  Mux6/1 -> Ankle Target/1
  Minus1/1 -> Mux2/1
  Low-Pass Filter (Discrete or Continuous)2/1 -> Hip Roll Target/1
  [swa] -> Mux6/1
  [swh_lat_a] -> Mux2/3
  [swh_lat_v] -> Product/1
  Product/1 -> Mux2/2
  Sign/1 -> Product/2
  Minus8/1 -> Mux3/1
  Mux3/1 -> Low-Pass Filter (Discrete or Continuous)1/1
  Low-Pass Filter (Discrete or Continuous)1/1 -> Hip Pitch Target/1
  Constant/1 -> Mux6/3, Mux6/2, Mux5/2, Mux3/2
  Switch/1 -> Mux5/3
  Constant1/1 -> Switch/1
  Constant2/1 -> Switch/3
  early/late/1 -> Switch/2
  Constant3/1 -> Mux3/3

== system ramadan_2022/Supraspinal Level/Subsystem/Swing Leg/Inverse Dynamics: Left Leg ==
  Desired Acceleration : Inport
  Enable : Inport  Port=2
  Inverse Dynamics : Subsystem
  Sensor Data from Body Layer : Subsystem
  Desired Torques : Outport
  Interaction Wrench : Outport  Port=2
  wires:
  Inverse Dynamics/1(" Desired Torques") -> Desired Torques/1
  Desired Acceleration/1 -> Inverse Dynamics/8(Desired Acceleration [rad/s^2])
  Sensor Data from Body Layer/4(" Rotation Trunk [rad]") -> Inverse Dynamics/4(Rotation Trunk [rad])
  Sensor Data from Body Layer/2(Joint Angle Velocities [rad/s]) -> Inverse Dynamics/2(Joint Angle Velocities [rad/s])
  Sensor Data from Body Layer/1(Joint Angles [rad]) -> Inverse Dynamics/1(Joint Angles [rad])
  Sensor Data from Body Layer/6(Rotation Velocity Trunk [rad/s]) -> Inverse Dynamics/6(Rotation Velocity Trunk [rad/s])
  Sensor Data from Body Layer/5(Trunk Position [m]) -> Inverse Dynamics/5(Trunk Position [m])
  Sensor Data from Body Layer/7(Trunk Velocity [m/s]) -> Inverse Dynamics/7(Trunk Velocity [m/s])
  Enable/1 -> Inverse Dynamics/Enable
  Inverse Dynamics/2(Interaction Wrench) -> Interaction Wrench/1
  Sensor Data from Body Layer/3(Joint Angle Accelerations [rad/s^2]) -> Inverse Dynamics/3(Joint  Acceleration [rad/s^2])

== system ramadan_2022/Supraspinal Level/Subsystem/Swing Leg/Inverse Dynamics: Right Leg ==
  Desired Acceleration : Inport
  Enable : Inport  Port=2
  Inverse Dynamics1 : Subsystem
  Sensor Data from Body Layer1 : Subsystem
  Desired Torques : Outport
  Interaction Wrench : Outport  Port=2
  wires:
  Inverse Dynamics1/1(" Desired Torques") -> Desired Torques/1
  Enable/1 -> Inverse Dynamics1/Enable
  Inverse Dynamics1/2(Interaction Wrench) -> Interaction Wrench/1
  Sensor Data from Body Layer1/1(Joint Angles [rad]) -> Inverse Dynamics1/1(Joint Angles [rad])
  Sensor Data from Body Layer1/2(Joint Angle Velocities [rad/s]) -> Inverse Dynamics1/2(Joint Angle Velocities [rad/s])
  Sensor Data from Body Layer1/3(Joint Angle Accelerations [rad/s^2]) -> Inverse Dynamics1/3(Joint  Acceleration [rad/s^2])
  Sensor Data from Body Layer1/4(" Rotation Trunk [rad]") -> Inverse Dynamics1/4(Rotation Trunk [rad])
  Sensor Data from Body Layer1/5(Trunk Position [m]) -> Inverse Dynamics1/5(Trunk Position [m])
  Sensor Data from Body Layer1/6(Rotation Velocity Trunk [rad/s]) -> Inverse Dynamics1/6(Rotation Velocity Trunk [rad/s])
  Sensor Data from Body Layer1/7(Trunk Velocity [m/s]) -> Inverse Dynamics1/7(Trunk Velocity [m/s])
  Desired Acceleration/1 -> Inverse Dynamics1/8(Desired Acceleration [rad/s^2])

== system ramadan_2022/Supraspinal Level/Subsystem/Compute positives forces that generate desired torque profiles/Left/sigmoid ==
  In1 : Inport
  Add : Sum
  Constant : Constant
  Constant1 : Constant
  Divide : Product  Inputs=*/
  Exp : Math  SaturateOnIntegerOverflow=on
  Gain : Gain  Gain=-1
  Out1 : Outport
  wires:
  Constant/1 -> Divide/1
  Constant1/1 -> Add/1
  In1/1 -> Gain/1
  Gain/1 -> Exp/1
  Exp/1 -> Add/2
  Add/1 -> Divide/2
  Divide/1 -> Out1/1

== system ramadan_2022/Supraspinal Level/Subsystem/Compute positives forces that generate desired torque profiles/Right/sigmoid ==
  In1 : Inport
  Add : Sum
  Constant : Constant
  Constant1 : Constant
  Divide : Product  Inputs=*/
  Exp : Math  SaturateOnIntegerOverflow=on
  Gain : Gain  Gain=-1
  Out1 : Outport
  wires:
  Constant/1 -> Divide/1
  Constant1/1 -> Add/1
  In1/1 -> Gain/1
  Gain/1 -> Exp/1
  Exp/1 -> Add/2
  Add/1 -> Divide/2
  Divide/1 -> Out1/1

== system ramadan_2022/Supraspinal Level/Subsystem/Stance Leg2/Stance Leg/Foot Orientation Left ==
  R Pelvis : Inport
  Coordinate Transformation Conversion1 : robotcorelib/Coordinate Transformation Conversion  InputRepresentation=Rotation Matrix  InputEulerSequence=ZYX  ShowTrVecInputPort=on  OutputRepresentation=Euler Angles  OutputEulerSequence=XYZ  ShowTrVecOutputPort=on  SimulateUsing=Code generation
      settings: SourceProductBaseCode=NV,RO,RR,UV
  Matrix Multiply : Product  Multiplication=Matrix(*)
  Selector2 : Selector  InputPortWidth=3  IndexOptions=Index vector (dialog)  Indices=[ 3]  OutputSizes=1
  Orientation Foot (Z) : Outport
  wires:
  Coordinate Transformation Conversion1/1 -> Selector2/1
  Matrix Multiply/1 -> Coordinate Transformation Conversion1/1
  Selector2/1 -> Orientation Foot (Z)/1
  R Pelvis/1 -> Matrix Multiply/1
  [RotationMatrixLeftFoot] -> Matrix Multiply/2

== system ramadan_2022/Supraspinal Level/Subsystem/Stance Leg2/Stance Leg/Foot Orientation Right ==
  R Pelvis : Inport
  Coordinate Transformation Conversion3 : robotcorelib/Coordinate Transformation Conversion  InputRepresentation=Rotation Matrix  InputEulerSequence=ZYX  ShowTrVecInputPort=on  OutputRepresentation=Euler Angles  OutputEulerSequence=XYZ  ShowTrVecOutputPort=on  SimulateUsing=Code generation
      settings: SourceProductBaseCode=NV,RO,RR,UV
  Matrix Multiply1 : Product  Multiplication=Matrix(*)
  Selector3 : Selector  InputPortWidth=3  IndexOptions=Index vector (dialog)  Indices=[ 3]  OutputSizes=1
  Foot Orientation (Z) : Outport
  wires:
  R Pelvis/1 -> Matrix Multiply1/1
  Selector3/1 -> Foot Orientation (Z)/1
  Coordinate Transformation Conversion3/1 -> Selector3/1
  [RotationMatrixRightFoot] -> Matrix Multiply1/2
  Matrix Multiply1/1 -> Coordinate Transformation Conversion3/1

== system ramadan_2022/Supraspinal Level/Subsystem/Stance Leg2/Stance Leg/Inverse Dynamics Left Leg ==
  Config [5] : Inport
  left/right : Inport  Port=2
  Task : Inport  Port=3
  PD Input : Inport  Port=4
  Left Leg Ball : Subsystem
  Low-Pass Filter (Discrete or Continuous) : eeGeneralControl/Low-Pass Filter (Discrete or Continuous)  K=1  T=0.01  B=150  A=-150  init_option=Inherited from block input  x0=0  Ts=-1
  Product : Product
  Selector4 : Selector  InputPortWidth=5  IndexOptions=Index vector (dialog)  Indices=[ 5 4 3 2]  OutputSizes=1
  Push-Off (Left) : Outport
  wires:
  Product/1 -> Selector4/1
  Selector4/1 -> Low-Pass Filter (Discrete or Continuous)/1
  Left Leg Ball/1(Push-Off Left (Ball)) -> Product/1
  Task/1 -> Left Leg Ball/2(Task)
  left/right/1 -> Product/2, Left Leg Ball/Enable
  Low-Pass Filter (Discrete or Continuous)/1 -> Push-Off (Left)/1
  Config [5]/1 -> Left Leg Ball/1(Config)
  PD Input/1 -> Left Leg Ball/3(PD Input)

== system ramadan_2022/Supraspinal Level/Subsystem/Stance Leg2/Stance Leg/Subsystem ==
  Config [5] : Inport
  left/right : Inport  Port=2
  Task : Inport  Port=3
  PD Input : Inport  Port=4
  Low-Pass Filter (Discrete or Continuous)1 : eeGeneralControl/Low-Pass Filter (Discrete or Continuous)  K=1  T=0.01  B=150  A=-150  init_option=Inherited from block input  x0=0  Ts=-1
  Product1 : Product
  Right Leg Ball : Subsystem
  Selector5 : Selector  InputPortWidth=5  IndexOptions=Index vector (dialog)  Indices=[ 5 4 3 2]  OutputSizes=1
  Push-Off (Right) : Outport
  wires:
  Selector5/1 -> Low-Pass Filter (Discrete or Continuous)1/1
  Low-Pass Filter (Discrete or Continuous)1/1 -> Push-Off (Right)/1
  Task/1 -> Right Leg Ball/2(Task)
  Right Leg Ball/1(Push-Off Right (Ball)) -> Product1/1
  Product1/1 -> Selector5/1
  Config [5]/1 -> Right Leg Ball/1(Config)
  left/right/1 -> Product1/2, Right Leg Ball/Enable
  PD Input/1 -> Right Leg Ball/3(PD)

== system ramadan_2022/Supraspinal Level/Subsystem/Swing Leg/Compute Acceleration Profiles with Minimal Jerk Approach/ Timer Phase 1 ==
  R : Inport
  Clock1 : Clock
  Clock3 : Clock
      settings: Decimation=4
  NOT : Logic  Operator=NOT  AllPortsSameDT=off  OutDataTypeStr=boolean
  Resettable Subsystem : Subsystem  TreatAsAtomicUnit=on
  Sum1 : Sum  Inputs=|+-  InputSameDT=on  SaturateOnIntegerOverflow=on  OutDataTypeStr=Inherit: Same as first input
  Switch2 : Switch  Criteria=u2 > Threshold  RndMeth=Zero
  t_passed : Outport  VectorParamsAs1DForOutWhenUnconnected=off
  wires:
  Clock1/1 -> Sum1/1
  Clock3/1 -> Switch2/3, Resettable Subsystem/1(In1)
  Sum1/1 -> t_passed/1
  R/1 -> NOT/1, Switch2/2
  Switch2/1 -> Sum1/2
  Resettable Subsystem/1(Out1) -> Switch2/1
  NOT/1 -> Resettable Subsystem/Enable

== system ramadan_2022/Supraspinal Level/Subsystem/Swing Leg/Compute Acceleration Profiles with Minimal Jerk Approach/ Timer Phase 2 ==
  R : Inport
  Clock1 : Clock
  Clock3 : Clock
      settings: Decimation=4
  NOT : Logic  Operator=NOT  AllPortsSameDT=off  OutDataTypeStr=boolean
  Resettable Subsystem : Subsystem  TreatAsAtomicUnit=on
  Sum1 : Sum  Inputs=|+-  InputSameDT=on  SaturateOnIntegerOverflow=on  OutDataTypeStr=Inherit: Same as first input
  Switch2 : Switch  Criteria=u2 > Threshold  RndMeth=Zero
  Out : Outport  VectorParamsAs1DForOutWhenUnconnected=off
  wires:
  Clock1/1 -> Sum1/1
  Clock3/1 -> Switch2/3, Resettable Subsystem/1(In1)
  Sum1/1 -> Out/1
  R/1 -> NOT/1, Switch2/2
  Switch2/1 -> Sum1/2
  Resettable Subsystem/1(Out1) -> Switch2/1
  NOT/1 -> Resettable Subsystem/Enable

== system ramadan_2022/Supraspinal Level/Subsystem/Swing Leg/Compute Acceleration Profiles with Minimal Jerk Approach/ Timer Phase 3 ==
  R : Inport
  Clock1 : Clock
  Clock3 : Clock
      settings: Decimation=4
  NOT : Logic  Operator=NOT  AllPortsSameDT=off  OutDataTypeStr=boolean
  Resettable Subsystem : Subsystem  TreatAsAtomicUnit=on
  Sum1 : Sum  Inputs=|+-  InputSameDT=on  SaturateOnIntegerOverflow=on  OutDataTypeStr=Inherit: Same as first input
  Switch2 : Switch  Criteria=u2 > Threshold  RndMeth=Zero
  t_passed : Outport  VectorParamsAs1DForOutWhenUnconnected=off
  wires:
  Clock1/1 -> Sum1/1
  Clock3/1 -> Switch2/3, Resettable Subsystem/1(In1)
  Sum1/1 -> t_passed/1
  R/1 -> NOT/1, Switch2/2
  Switch2/1 -> Sum1/2
  Resettable Subsystem/1(Out1) -> Switch2/1
  NOT/1 -> Resettable Subsystem/Enable

== system ramadan_2022/Supraspinal Level/Subsystem/Swing Leg/Compute Acceleration Profiles with Minimal Jerk Approach/ Timer Phase 4 ==
  R : Inport
  Clock1 : Clock
  Clock3 : Clock
      settings: Decimation=4
  NOT : Logic  Operator=NOT  AllPortsSameDT=off  OutDataTypeStr=boolean
  Resettable Subsystem : Subsystem  TreatAsAtomicUnit=on
  Sum1 : Sum  Inputs=|+-  InputSameDT=on  SaturateOnIntegerOverflow=on  OutDataTypeStr=Inherit: Same as first input
  Switch2 : Switch  Criteria=u2 > Threshold  RndMeth=Zero
  t_passed : Outport  VectorParamsAs1DForOutWhenUnconnected=off
  wires:
  Clock1/1 -> Sum1/1
  Clock3/1 -> Switch2/3, Resettable Subsystem/1(In1)
  Sum1/1 -> t_passed/1
  R/1 -> NOT/1, Switch2/2
  Switch2/1 -> Sum1/2
  Resettable Subsystem/1(Out1) -> Switch2/1
  NOT/1 -> Resettable Subsystem/Enable

== system ramadan_2022/Supraspinal Level/Subsystem/Swing Leg/Compute Acceleration Profiles with Minimal Jerk Approach/Minimal jerk Ankle ==
  T_tot : Inport
  t_passed : Inport  Port=2
  "x0, dx0, ddx0" : Inport  Port=3
  "xT, dxT, ddxT" : Inport  Port=4
  Compare To Constant : simulink/Logic and Bit Operations/Compare To Constant  relop=>=  const=mParams.control.timelimit  OutDataTypeStr=boolean  ZeroCross=off
  Constant : Constant  Value=mParams.control.timelimit
  Constant1 : Constant  Value=0
  Demux : Demux  Outputs=3
  Demux1 : Demux  Outputs=3
  Enabled Subsystem : Subsystem  TreatAsAtomicUnit=on
  Minimal Jerk : Subsystem
  Minimal Jerk Parameters [Movellan] : Subsystem
  Minus : Sum  Inputs=+-
  Minus1 : Sum  Inputs=+-
  Switch : Switch
  jerk : Outport
  wires:
  Minimal Jerk/1(j(t)) -> jerk/1
  T_tot/1 -> Minus/1
  t_passed/1 -> Minus/2
  Constant1/1 -> Switch/1
  Demux/1 -> Minimal Jerk Parameters [Movellan]/1(x0)
  Demux/2 -> Minimal Jerk Parameters [Movellan]/2(dx0)
  Demux/3 -> Minimal Jerk Parameters [Movellan]/3(ddx0)
  Demux1/1 -> Minimal Jerk Parameters [Movellan]/4(xT)
  "x0, dx0, ddx0"/1 -> Demux/1
  Demux1/2 -> Minimal Jerk Parameters [Movellan]/5(dxT)
  "xT, dxT, ddxT"/1 -> Demux1/1
  Demux1/3 -> Minimal Jerk Parameters [Movellan]/6(ddxT)
  Minimal Jerk Parameters [Movellan]/1(a) -> Enabled Subsystem/1(In1)
  Minus/1 -> Compare To Constant/1, Minus1/2, Minimal Jerk Parameters [Movellan]/7(T)
  Enabled Subsystem/1(Out1) -> Minimal Jerk/2(a [6x1])
  Compare To Constant/1 -> Switch/2, Enabled Subsystem/Enable
  Constant/1 -> Minus1/1
  Minus1/1 -> Switch/3
  Switch/1 -> Minimal Jerk/1(t)

== system ramadan_2022/Supraspinal Level/Subsystem/Swing Leg/Compute Acceleration Profiles with Minimal Jerk Approach/Minimal jerk Hip Pitch ==
  T_tot : Inport
  t_passed : Inport  Port=2
  "x0, dx0, ddx0" : Inport  Port=3
  "xT, dxT, ddxT" : Inport  Port=4
  Compare To Constant : simulink/Logic and Bit Operations/Compare To Constant  relop=>=  const=mParams.control.timelimit  OutDataTypeStr=boolean  ZeroCross=off
  Constant : Constant  Value=mParams.control.timelimit
  Constant1 : Constant  Value=0
  Demux : Demux  Outputs=3
  Demux1 : Demux  Outputs=3
  Enabled Subsystem : Subsystem  TreatAsAtomicUnit=on
  Minimal Jerk : Subsystem
  Minimal Jerk Parameters [Movellan] : Subsystem
  Minus : Sum  Inputs=+-
  Minus1 : Sum  Inputs=+-
  Switch : Switch
  jerk : Outport
  wires:
  Minimal Jerk/1(j(t)) -> jerk/1
  T_tot/1 -> Minus/1
  t_passed/1 -> Minus/2
  Constant1/1 -> Switch/1
  Demux/1 -> Minimal Jerk Parameters [Movellan]/1(x0)
  Demux/2 -> Minimal Jerk Parameters [Movellan]/2(dx0)
  Demux/3 -> Minimal Jerk Parameters [Movellan]/3(ddx0)
  Demux1/1 -> Minimal Jerk Parameters [Movellan]/4(xT)
  "x0, dx0, ddx0"/1 -> Demux/1
  Demux1/2 -> Minimal Jerk Parameters [Movellan]/5(dxT)
  "xT, dxT, ddxT"/1 -> Demux1/1
  Demux1/3 -> Minimal Jerk Parameters [Movellan]/6(ddxT)
  Minimal Jerk Parameters [Movellan]/1(a) -> Enabled Subsystem/1(In1)
  Minus/1 -> Compare To Constant/1, Minus1/2, Minimal Jerk Parameters [Movellan]/7(T)
  Enabled Subsystem/1(Out1) -> Minimal Jerk/2(a [6x1])
  Compare To Constant/1 -> Switch/2, Enabled Subsystem/Enable
  Constant/1 -> Minus1/1
  Minus1/1 -> Switch/3
  Switch/1 -> Minimal Jerk/1(t)
